simulink model "RS232ex4"  (Simulink 5.0)
settings: Solver=ode3  StartTime=0.0  StopTime=5  FixedStep=1  RelTol=1e-3
libraries: RS232 x4
settings Model: LastModifiedBy=leo

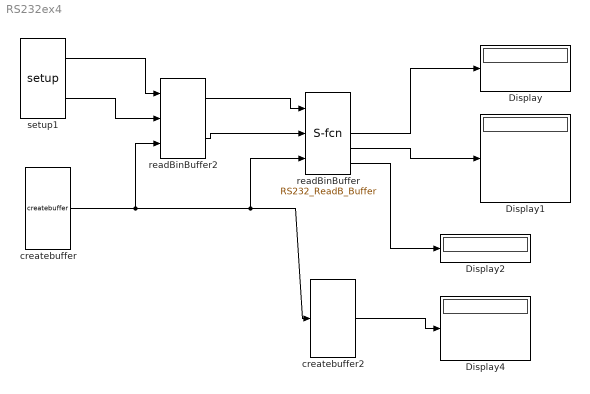
== system RS232ex4 ==
  Display{,1..2,4} (4 alike) : Display
  createbuffer : RS232/createbuffer  minbuffsize=128  sampletime=-1
  createbuffer2 : RS232/createbuffer2  sampletime=-1
  readBinBuffer : S-Function  FunctionName=RS232_ReadB_Buffer  Parameters=fmtString,sampTime,allocstep  mask(readbinbuffer){fmtString=2i1,3u4,1d8, sampTime=-1, allocstep=512}
      mask prompts: fmtString "Format String"; sampTime "Sample time"; allocstep "Allocation Step"
      mask help: RS232 Read Binary Buffer
      mask Help: RS232 Read Binary Buffer
      mask Display: disp('RS232\nRead\nBinary\nBuffer');
  readBinBuffer2 : RS232/readBinBuffer2  synchsize=2  mask=0xffff  value=0x0209  sampTime=-1  allocstep=512
  setup1 : RS232/setup  port=COM1  baudrate=38400  databit=8  stopbit=1  parity=None
  wires:
  createbuffer/1 -> readBinBuffer2/3, readBinBuffer/3, createbuffer2/1
  setup1/2 -> readBinBuffer2/2
  setup1/1 -> readBinBuffer2/1
  readBinBuffer2/1 -> readBinBuffer/1
  readBinBuffer2/2 -> readBinBuffer/2
  readBinBuffer/5 -> Display2/1
  createbuffer2/1 -> Display4/1
  readBinBuffer/3 -> Display/1
  readBinBuffer/4 -> Display1/1
